simulink model "ipd_lifting_sim"  (R2024a)
settings: Solver=VariableStepAuto  StartTime=0.0  StopTime=5  RelTol=1e-3
values from neighbouring files (symbols this model uses):
  A = [0,  1 ... (first row only)    [ipd_lifted_regulator.m]
  B = [0 ... (first row only)    [ipd_lifted_regulator.m]
  C = eye(2)    [ipd_lifted_regulator.m]
  D = [0 ... (first row only)    [ipd_lifted_regulator.m]
  h = 0.02    [cart_ipd_control.m]    (also in ipd_lifted_regulator.m = 0.06)
  t_sim = 0.001    [cart_ipd_control.m]    (also in ipd_lifted_regulator.m)
  x0 = 0.0    (= 0)    [cart_ipd_control.m]    (also in ipd_lifted_regulator.m = [1.5)
undefined symbols (not defined in the file or in its folder): K, Ks
settings Model: Creator=Fumiya Matsuzaki  LastModifiedBy=Fumiya Matsuzaki

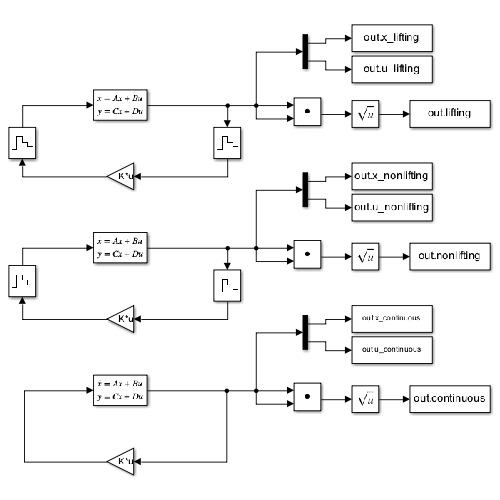
[thumbnail: Simulink's stored preview of the top-level diagram]
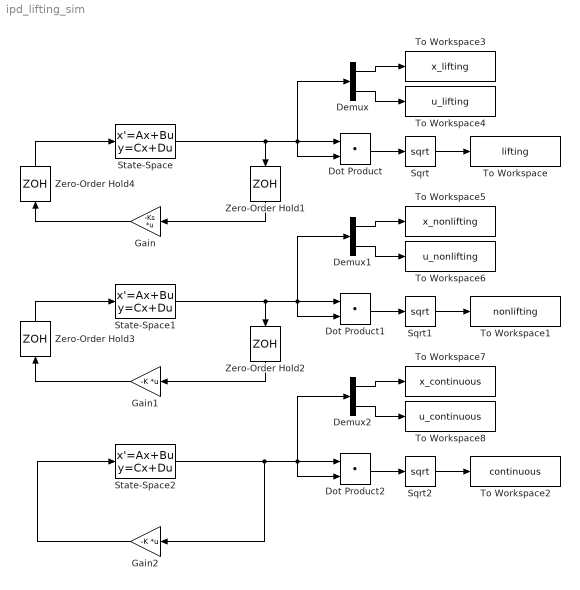
== system ipd_lifting_sim ==
  Demux : Demux  Outputs=2
  Demux1 : Demux  Outputs=2
  Demux2 : Demux  Outputs=2
  Dot Product : DotProduct  OutDataTypeStr=Inherit: Inherit via internal rule
  Dot Product1 : DotProduct  OutDataTypeStr=Inherit: Inherit via internal rule
  Dot Product2 : DotProduct  OutDataTypeStr=Inherit: Inherit via internal rule
  Gain : Gain  Gain=-Ks  Multiplication=Matrix(K*u)
  Gain1 : Gain  Gain=-K  Multiplication=Matrix(K*u)
  Gain2 : Gain  Gain=-K  Multiplication=Matrix(K*u)
  Sqrt : Sqrt
  Sqrt1 : Sqrt
  Sqrt2 : Sqrt
  State-Space : StateSpace  A=A  B=B  C=C  D=D  InitialCondition=x0
  State-Space1 : StateSpace  A=A  B=B  C=C  D=D  InitialCondition=x0
  State-Space2 : StateSpace  A=A  B=B  C=C  D=D  InitialCondition=x0
  To Workspace : ToWorkspace  VariableName=lifting  SampleTime=-1
  To Workspace1 : ToWorkspace  VariableName=nonlifting  SampleTime=-1
  To Workspace2 : ToWorkspace  VariableName=continuous  SampleTime=-1
  To Workspace3 : ToWorkspace  VariableName=x_lifting  SampleTime=-1
  To Workspace4 : ToWorkspace  VariableName=u_lifting  SampleTime=-1
  To Workspace5 : ToWorkspace  VariableName=x_nonlifting  SampleTime=-1
  To Workspace6 : ToWorkspace  VariableName=u_nonlifting  SampleTime=-1
  To Workspace7 : ToWorkspace  VariableName=x_continuous  SampleTime=-1
  To Workspace8 : ToWorkspace  VariableName=u_continuous  SampleTime=-1
  Zero-Order Hold1 : ZeroOrderHold  SampleTime=h
  Zero-Order Hold2 : ZeroOrderHold  SampleTime=h
  Zero-Order Hold3 : ZeroOrderHold  SampleTime=t_sim
  Zero-Order Hold4 : ZeroOrderHold  SampleTime=t_sim
  wires:
  State-Space/1 -> Demux/1, Dot Product/2, Dot Product/1, Zero-Order Hold1/1
  Gain/1 -> Zero-Order Hold4/1
  Gain1/1 -> Zero-Order Hold3/1
  Gain2/1 -> State-Space2/1
  Sqrt/1 -> To Workspace/1
  Dot Product/1 -> Sqrt/1
  Sqrt1/1 -> To Workspace1/1
  Dot Product1/1 -> Sqrt1/1
  Dot Product2/1 -> Sqrt2/1
  Sqrt2/1 -> To Workspace2/1
  Zero-Order Hold2/1 -> Gain1/1
  Zero-Order Hold3/1 -> State-Space1/1
  Zero-Order Hold1/1 -> Gain/1
  Zero-Order Hold4/1 -> State-Space/1
  Demux/1 -> To Workspace3/1
  Demux/2 -> To Workspace4/1
  Demux1/1 -> To Workspace5/1
  State-Space1/1 -> Dot Product1/2, Demux1/1, Dot Product1/1, Zero-Order Hold2/1
  Demux1/2 -> To Workspace6/1
  Demux2/1 -> To Workspace7/1
  State-Space2/1 -> Dot Product2/2, Demux2/1, Dot Product2/1, Gain2/1
  Demux2/2 -> To Workspace8/1
